simulink model "cpu2"  (R2024b)
settings: Solver=FixedStepAuto  StartTime=0.0  StopTime=Inf  FixedStep=0.0001  RelTol=1e-3  EnableMultiTasking=on
undefined symbols (not defined in the file or in its folder): C28x, CPU1, CPU2
libraries: c2837xDlib x3
settings Model: ExtModeTrigDuration=8  Creator=lenovo  LastModifiedBy=chaiy
settings OptimizationCC: DefaultUnderspecifiedDataType=single  EnhancedBackFolding=on  PassReuseOutputArgsAs=Individual arguments  MaxStackSize=1024  OptimizeBlockOrder=speed  DifferentSizesBufferReuse=on  OptimizationCustomize=off  DenormalBehavior=FlushToZero  EfficientTunableParamExpr=on
settings DebuggingCC: ParameterTunabilityLossMsg=error
settings HardwareCC: ProdBitPerChar=16  ProdBitPerInt=16  ProdBitPerPointer=32  ProdBitPerSizeT=32  ProdBitPerPtrDiffT=32  ProdLargestAtomicInteger=Integer  ProdLargestAtomicFloat=None  ProdWordSize=16  ProdLongLongMode=on  ProdHWDeviceType=Texas Instruments->C2000
settings ModelReferenceCC: EnableRefExpFcnMdlSchedulingChecks=on  ModelReferenceNumInstancesAllowed=Single
settings SFSimCC: MATLABDynamicMemAlloc=off
settings RTWCC: Description=Embedded Coder  SystemTargetFile=ert.tlc  HardwareBoard=TI Delfino F28379D LaunchPad  TemplateMakefile=ert_default_tmf  Toolchain=Texas Instruments Code Composer Studio (C2000)  CodeExecutionProfiling=on  CodeProfilingSaveOptions=MetricsOnly  CodeProfilingInstrumentation=detailed  GPUComputeCapability=3.5
settings CodeAppCC: ForceParamTrailComments=on  IgnoreCustomStorageClasses=off  MaxIdLength=95  OperatorAnnotations=on  SimulinkDataObjDesc=on  SFDataObjDesc=on  InsertBlockDesc=on
settings ERTTargetCC: CodeReplacementLibrary=TI C28x  SupportContinuousTime=on  ExtModeTransport=4  ExtModeStaticAlloc=on  ExtModeAutomaticAllocSize=off  ExtModeStaticAllocSize=10000  ExtModeMexFile=ext_xcp  ExtModeIntrfLevel=Level2 - Open  InlinedParameterPlacement=Hierarchical  DynamicArrayContainerType=coder::array

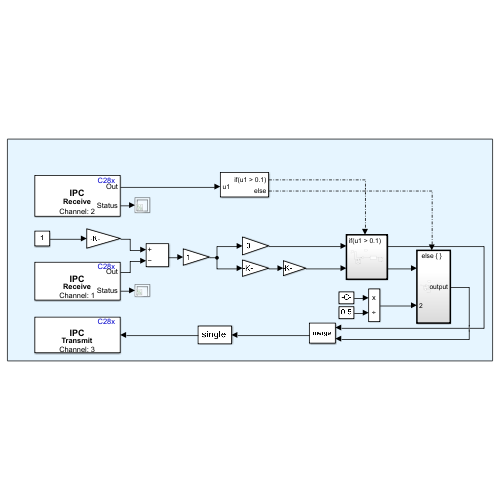
[thumbnail: Simulink's stored preview of the top-level diagram]
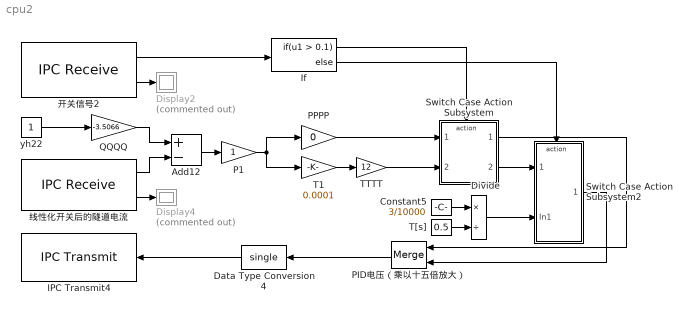
== system cpu2 ==
  Add12 : Sum  Inputs=+-
  Constant5 : Constant  Value=3/10000  SampleTime=0.0001
  Data Type Conversion4 : DataTypeConversion  OutDataTypeStr=single  SaturateOnIntegerOverflow=off  RndMeth=Floor
  Display2 : Display  Commented=on
  Display4 : Display  Commented=on
  Divide : Product  Inputs=*/
  IPC Transmit4 : c2837xDlib/IPC Transmit  blkParamProc=F2837x  SelectDestination=C28x (CPU1/CPU2)  SelectChannel=3  EnableBlocking=off
  If : If  IfExpression=u1 > 0.1
  P1 : Gain
  PID电压（乘以十五倍放大） : Merge
  PPPP : Gain  Gain=0
  QQQQ : Gain  Gain=-3.5066
  Switch Case Action Subsystem : Subsystem  TreatAsAtomicUnit=on
  Switch Case Action Subsystem2 : Subsystem  TreatAsAtomicUnit=on
  T1 : Gain  Gain=0.0001
  TTTT : Gain  Gain=12
  T[s] : Constant  Value=0.5  SampleTime=0.0001
  yh22 : Constant  SampleTime=0.0001
  开关信号2 : c2837xDlib/IPC Receive  blkParamProc=F2837x  SelectSource=C28x (CPU1/CPU2)  SelectChannel=2  DataType=single  DataLength=1  EnableBlocking=off  SampleTime=0.0001
  线性化开关后的隧道电流 : c2837xDlib/IPC Receive  blkParamProc=F2837x  SelectSource=C28x (CPU1/CPU2)  SelectChannel=1  DataType=single  DataLength=1  EnableBlocking=off  SampleTime=0.0001
  wires:
  If/1 -> Switch Case Action Subsystem/Action
  开关信号2/1 -> If/1
  If/2 -> Switch Case Action Subsystem2/Action
  线性化开关后的隧道电流/1 -> Add12/2
  Switch Case Action Subsystem/1(output) -> PID电压（乘以十五倍放大）/1
  Switch Case Action Subsystem2/1(output) -> PID电压（乘以十五倍放大）/2
  Switch Case Action Subsystem/2(u_sum1) -> Switch Case Action Subsystem2/1(累减器的初始状态)
  PID电压（乘以十五倍放大）/1 -> Data Type Conversion4/1
  P1/1 -> T1/1, PPPP/1
  QQQQ/1 -> Add12/1
  Add12/1 -> P1/1
  TTTT/1 -> Switch Case Action Subsystem/2(积分控制1)
  开关信号2/2 -> Display2/1
  PPPP/1 -> Switch Case Action Subsystem/1(比例控制1)
  线性化开关后的隧道电流/2 -> Display4/1
  T[s]/1 -> Divide/2
  T1/1 -> TTTT/1
  Divide/1 -> Switch Case Action Subsystem2/2(In1)
  Constant5/1 -> Divide/1
  Data Type Conversion4/1 -> IPC Transmit4/1
  yh22/1 -> QQQQ/1

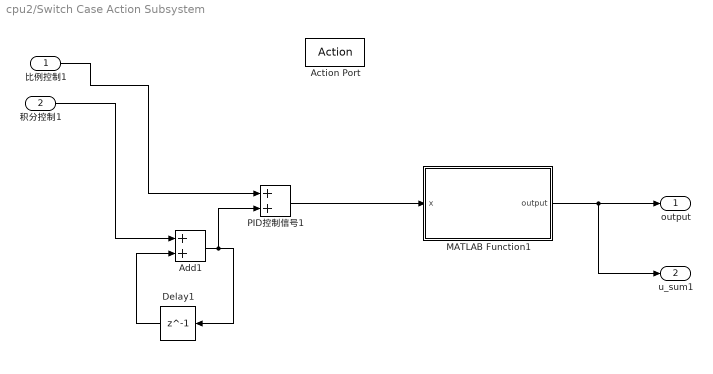
== system cpu2/Switch Case Action Subsystem ==
  比例控制1 : Inport
  积分控制1 : Inport  Port=2
  Action Port : ActionPort  InitializeStates=reset  ActionPortLabel=if(u1 > 0.1)
  Add1 : Sum
  Delay1 : Delay  DelayLength=1  SampleTime=0.0001
  MATLAB Function1 : MATLAB Function  TreatAsAtomicUnit=on
  PID控制信号1 : Sum
  output : Outport
  u_sum1 : Outport  Port=2
  wires:
  比例控制1/1 -> PID控制信号1/1
  Add1/1 -> Delay1/1, PID控制信号1/2
  积分控制1/1 -> Add1/1
  Delay1/1 -> Add1/2
  PID控制信号1/1 -> MATLAB Function1/1(x)
  MATLAB Function1/1(output) -> u_sum1/1, output/1

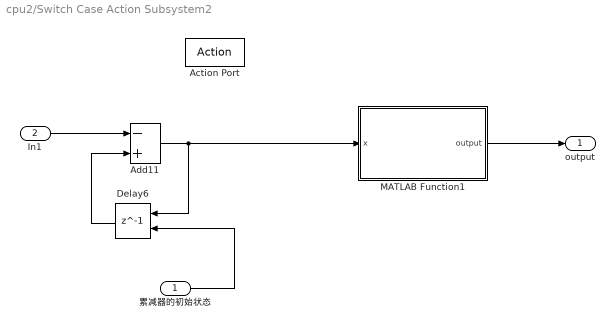
== system cpu2/Switch Case Action Subsystem2 ==
  累减器的初始状态 : Inport
  In1 : Inport  Port=2
  Action Port : ActionPort  InitializeStates=reset  PropagateVarSize=During execution  ActionPortLabel=else
  Add11 : Sum  Inputs=-+
  Delay6 : Delay  DelayLength=1  InitialConditionSource=Input port  SampleTime=0.0001
      settings: InputPortMap=u0,p4
  MATLAB Function1 : MATLAB Function  TreatAsAtomicUnit=on
  output : Outport
  wires:
  累减器的初始状态/1 -> Delay6/2
  In1/1 -> Add11/1
  Delay6/1 -> Add11/2
  MATLAB Function1/1(output) -> output/1
  Add11/1 -> MATLAB Function1/1(x), Delay6/1

== matlab function cpu2/Switch Case Action Subsystem/MATLAB Function1 ==
  data: x input; output output
function output = limit_input(x)

    output = min(x, 3);

end

== matlab function cpu2/Switch Case Action Subsystem2/MATLAB Function1 ==
  data: x input; output output
function output = limit_min_zero(x)

    output = max(x, 0);
end
